simulink model "model_Tp0bb"  (R2018a)
settings: Solver=ode45  StartTime=0.0  StopTime=5  MaxStep=1e-3  RelTol=1e-3
values from neighbouring files (symbols this model uses):
  J = (Tm*KN^2)/Ra    (= 0.00790540540541)    [Tp0.m]
  KN = Kt    (= 0.5)    [Tp0.m]
  Kpn = KN*(TM/(2*Ta)-1)    (= 0.222222222222)    [Tp0.m]
  La = Te*Ra    (= 0.0014985)    [Tp0.m]
  Ra = 0.37    [Tp0.m]
  Tc = 15    [Tp0.m]
  Tin = 4*Ta*(1-2*Ta/(TM))    (= 0.00498461538462)    [Tp0.m]
  wref = 392    [Tp0.m]
libraries: simulink x3
settings Model: Creator=Lac User  LastModifiedBy=matia
settings DataIOCC: SaveFormat=StructureWithTime  ReturnWorkspaceOutputs=on
settings OptimizationCC: LifeSpan=inf
settings DebuggingCC: SFExecutionAtInitializationDiag=none
settings HardwareCC: ProdBitPerSizeT=32  ProdBitPerPtrDiffT=32  ProdWordSize=32  ProdHWDeviceType=Specified
settings SFSimCC: SimUseLocalCustomCode=on
settings RTWCC: RTWUseLocalCustomCode=on
settings CodeAppCC: StateflowObjectComments=on

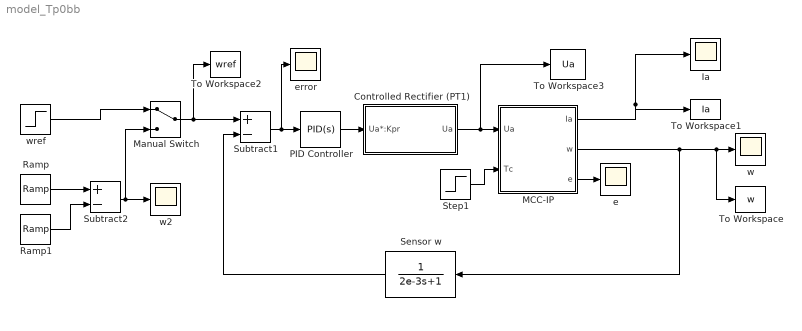
== system model_Tp0bb ==
  Controlled Rectifier (PT1) : Subsystem  mask(Controlled Rectifier (PT1)){Tpr=0.2e-2, Kpr=1}
      mask prompts: Tpr "Controlled Rectifier Integral Gain:"; Kpr "Controlled Rectifier Gain:"
      mask Display:
      | plot([0.45 0.8 0.8 0.45 0.45],[0.15 0.15 .85 .85 0.15])
      | plot(0.42+0.5*(0.1:0.02:0.7),0.2+0.3*log(1:0.2:7))
  Ia : Scope
  MCC-IP : Subsystem
  Manual Switch : ManualSwitch
  PID Controller : simulink/Continuous/PID Controller  Controller=PID  TimeDomain=Continuous-time  SampleTime=-1  IntegratorMethod=Forward Euler  FilterMethod=Forward Euler  Form=Parallel  UseFilter=on  ControllerParametersSource=internal  P=Kpn  I=Kpn/Tin  D=0  N=100  InitialConditionSource=internal  InitialConditionForIntegrator=0  InitialConditionForFilter=0  ExternalReset=none  LimitOutput=off  UpperSaturationLimit=inf  LowerSaturationLimit=-inf  LinearizeAsGain=on  AntiWindupMode=none  Kb=1  TrackingMode=off  Kt=1  PParamMin=[]  PParamMax=[]  IParamMin=[]  IParamMax=[]  DParamMin=[]  DParamMax=[]  NParamMin=[]  NParamMax=[]  KbParamMin=[]  KbParamMax=[]  KtParamMin=[]  KtParamMax=[]  POutMin=[]  POutMax=[]  IOutMin=[]  IOutMax=[]  DOutMin=[]  DOutMax=[]  NOutMin=[]  NOutMax=[]  KbOutMin=[]  KbOutMax=[]  KtOutMin=[]  KtOutMax=[]  IntegratorOutMin=[]  IntegratorOutMax=[]  FilterOutMin=[]  FilterOutMax=[]  SumOutMin=[]  SumOutMax=[]  SumI1OutMin=[]  SumI1OutMax=[]  SumI2OutMin=[]  SumI2OutMax=[]  SumI3OutMin=[]  SumI3OutMax=[]  SumDOutMin=[]  SumDOutMax=[]  SaturationOutMin=[]  SaturationOutMax=[]  IntegratorContinuousStateAttributes=''  IntegratorStateMustResolveToSignalObject=off  IntegratorRTWStateStorageClass=Auto  FilterContinuousStateAttributes=''  FilterStateMustResolveToSignalObject=off  FilterRTWStateStorageClass=Auto  DifferentiatorICPrevScaledInput=0  DifferentiatorOutMin=[]  DifferentiatorOutMax=[]  FilterDiffOutCoefMin=[]  FilterDiffOutCoefMax=[]  SumDenOutMin=[]  SumDenOutMax=[]  SumNumOutMin=[]  SumNumOutMax=[]  ReciprocalOutMin=[]  ReciprocalOutMax=[]  DivideOutMin=[]  DivideOutMax=[]  TunerSelectOption=Transfer Function Based (PID Tuner App)
  Ramp : simulink/Sources/Ramp  slope=wref*4  start=0  InitialOutput=0
  Ramp1 : simulink/Sources/Ramp  slope=wref*4  start=0.25  InitialOutput=0
  Sensor w : TransferFcn  Denominator=[2e-3 1]
  Step1 : Step  Time=2.5  After=Tc  SampleTime=0
  Subtract1 : Sum  Inputs=+-
  Subtract2 : Sum  Inputs=+-
  To Workspace : ToWorkspace  VariableName=w  SampleTime=-1
  To Workspace1 : ToWorkspace  VariableName=Ia  SampleTime=-1
  To Workspace2 : ToWorkspace  VariableName=wref  SampleTime=-1
  To Workspace3 : ToWorkspace  VariableName=Ua  SampleTime=-1
  e : Scope
  error : Scope
  w : Scope
  w2 : Scope
  wref : Step  Time=0  After=wref  SampleTime=0
  wires:
  MCC-IP/1(Ia) -> To Workspace1/1, Ia/1
  MCC-IP/2(w) -> Sensor w/1, To Workspace/1, w/1
  MCC-IP/3(e) -> e/1
  Subtract1/1 -> error/1, PID Controller/1
  Step1/1 -> MCC-IP/2(Tc)
  Subtract2/1 -> Manual Switch/2, w2/1
  Ramp/1 -> Subtract2/1
  Ramp1/1 -> Subtract2/2
  wref/1 -> Manual Switch/1
  Manual Switch/1 -> To Workspace2/1, Subtract1/1
  PID Controller/1 -> Controlled Rectifier (PT1)/1(Ua*:Kpr)
  Controlled Rectifier (PT1)/1(Ua) -> To Workspace3/1, MCC-IP/1(Ua)
  Sensor w/1 -> Subtract1/2

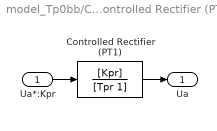
== system model_Tp0bb/Controlled Rectifier (PT1) ==
  Ua*:Kpr : Inport
  Controlled Rectifier (PT1) : TransferFcn  Numerator=[Kpr]  Denominator=[Tpr 1]
  Ua : Outport
  wires:
  Controlled Rectifier (PT1)/1 -> Ua/1
  Ua*:Kpr/1 -> Controlled Rectifier (PT1)/1

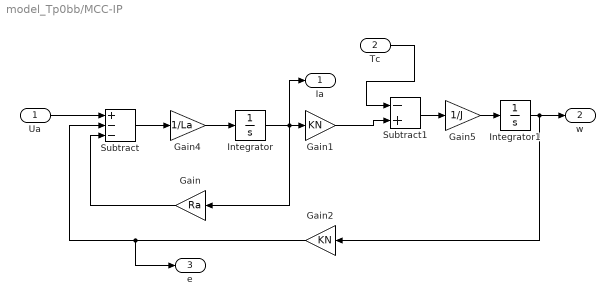
== system model_Tp0bb/MCC-IP ==
  Ua : Inport
  Tc : Inport  Port=2
  Gain : Gain  Gain=Ra
  Gain1 : Gain  Gain=KN
  Gain2 : Gain  Gain=KN
  Gain4 : Gain  Gain=1/La
  Gain5 : Gain  Gain=1/J
  Integrator : Integrator
  Integrator1 : Integrator
  Subtract : Sum  Inputs=+--
  Subtract1 : Sum  Inputs=-+
  Ia : Outport
  w : Outport  Port=2
  e : Outport  Port=3
  wires:
  Subtract1/1 -> Gain5/1
  Gain4/1 -> Integrator/1
  Gain1/1 -> Subtract1/2
  Subtract/1 -> Gain4/1
  Integrator1/1 -> w/1, Gain2/1
  Integrator/1 -> Ia/1, Gain/1, Gain1/1
  Gain2/1 -> e/1, Subtract/2
  Gain/1 -> Subtract/3
  Gain5/1 -> Integrator1/1
  Ua/1 -> Subtract/1
  Tc/1 -> Subtract1/1
